simulink model "lab4m3"  (R2018a)
settings: Solver=ode4  StartTime=0.0  StopTime=10.0  FixedStep=1e-2  RelTol=1e-3
values from neighbouring files (symbols this model uses):
  bot = botl(f,:)    [MarcinGrzybS.m]
  top = topl(f,:)    [MarcinGrzybS.m]
settings Model: Creator=nicra  LastModifiedBy=nicra

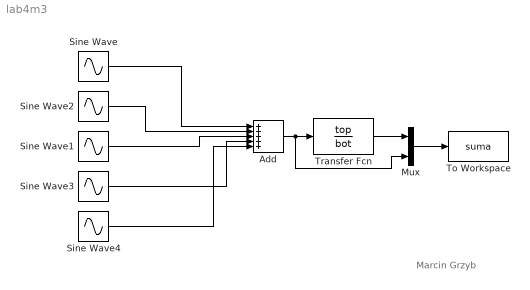
== system lab4m3 ==
  note: Marcin Grzyb
  Add : Sum  Inputs=+++++
  Mux : Mux  Inputs=2
  Sine Wave : Sin  Amplitude=2  Frequency=0.001  Phase=1  SampleTime=0
  Sine Wave1 : Sin  Frequency=30  Phase=2  SampleTime=0
  Sine Wave2 : Sin  Amplitude=3  Phase=5  SampleTime=0
  Sine Wave3 : Sin  Amplitude=2  Frequency=0.01  Phase=1  SampleTime=0
  Sine Wave4 : Sin  Amplitude=4  Frequency=5  SampleTime=0
  To Workspace : ToWorkspace  VariableName=suma  SaveFormat=Timeseries  SampleTime=-1
  Transfer Fcn : TransferFcn  Numerator=top  Denominator=bot
  wires:
  Sine Wave/1 -> Add/1
  Sine Wave2/1 -> Add/2
  Sine Wave1/1 -> Add/3
  Sine Wave3/1 -> Add/4
  Sine Wave4/1 -> Add/5
  Add/1 -> Mux/2, Transfer Fcn/1
  Mux/1 -> To Workspace/1
  Transfer Fcn/1 -> Mux/1
